simulink model "Diagramas_pruebas_modelo_definitivo"  (R2023b)
settings: Solver=VariableStepAuto  StartTime=0.0  StopTime=1.9  MaxStep=1e-5  RelTol=1e-3
values from neighbouring files (symbols this model uses):
  alpha_cu = 3.9 * 10^(-3)    (= 0.0039)    [parametros.m]
  b_eq = 2.1944e-5    (= 2.1944e-05)    [diagrama_polos_y_ceros_LTI.m]    (also in main.m = 2.19444444444e-05; parametros.m = 2.21527777778e-05)
  C_ts = 0.818    [parametros.m]
  J_eq = 1.9785e-5    (= 1.9785e-05)    [diagrama_polos_y_ceros_LTI.m]    (also in main.m = 1.97847222222e-05; parametros.m = 1.97847222222e-05)
  k_l = 0.25    [main.m]    (also in parametros.m)
  L_d = 6.6    [main.m]    (also in parametros.m = 0.0066)
  L_q = 5.8e-3    (= 0.0058)    [diagrama_polos_y_ceros_LTI.m]    (also in main.m = 5.8; parametros.m; variacion_de_parametros.m)
  P_p = 3    [Simulacion_Temporal_corrientesytensiones.m]    (also in diagrama_polos_y_ceros_LTI.m; main.m; parametros.m; variacion_de_parametros.m)
  r = 120.0    (= 120)    [diagrama_polos_y_ceros_LTI.m]    (also in main.m; parametros.m)
  R_sref = 1.02    [parametros.m]
  R_tsamb = 146.7    [parametros.m]
  T_sref = 20    [parametros.m]
libraries: SignalEditorBlockLib x2
settings Model: Creator=nicol  LastModifiedBy=Julya

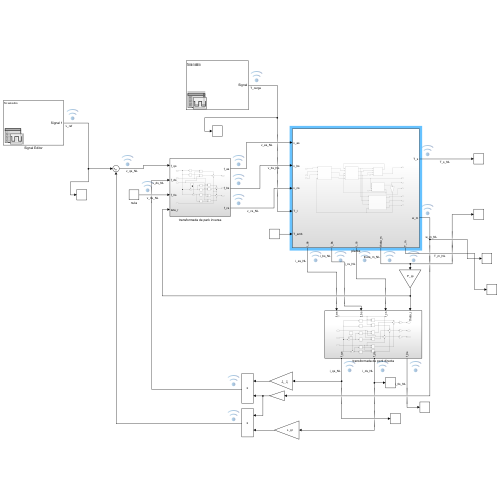
[thumbnail: Simulink's stored preview of the top-level diagram]
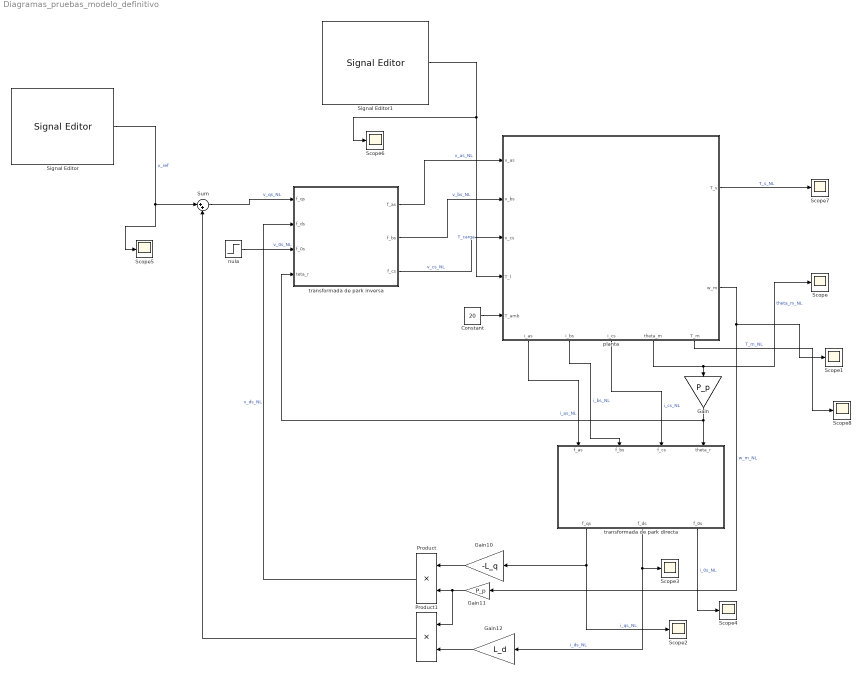
== system Diagramas_pruebas_modelo_definitivo ==
  Constant : Constant  Value=20
  Gain : Gain  Gain=P_p
  Gain10 : Gain  Gain=-L_q
  Gain11 : Gain  Gain=P_p
  Gain12 : Gain  Gain=L_d
  Product : Product
  Product1 : Product
  Scope{,1..8} (9 alike) : Scope
  Signal Editor : SignalEditorBlockLib/Signal Editor  FileName=V_qs_ref.mat  ActiveScenario=Scenario  ActiveSignal=Signal 1  IsBus=off  OutputBusObjectStr=Bus: BusObject  SampleTime=0  Interpolate=off  ZeroCross=off  OutputAfterFinalValue=Setting to zero  Unit=inherit  PreserveSignalName=on  ApplySigPropsToAllScenarios=on  ApplySigPropsToAllSignals=off
  Signal Editor1 : SignalEditorBlockLib/Signal Editor  FileName=Pulso_Torque_Carga.mat  ActiveScenario=Scenario  ActiveSignal=Signal  IsBus=off  OutputBusObjectStr=Bus: BusObject  SampleTime=0  Interpolate=off  ZeroCross=off  OutputAfterFinalValue=Setting to zero  Unit=inherit  PreserveSignalName=on  ApplySigPropsToAllScenarios=on  ApplySigPropsToAllSignals=off
  Sum : Sum  Inputs=|++
  nula : Step  Time=0  After=0  SampleTime=0
  planta : Subsystem
      settings: PortSchema="{\"entries\":[{\"content\":{\"sides\":[{\"content\":{\"connectorIds\":[\"In1\",\"In2\",\"In3\",\"In4\",\"In5\"]},\"type\":\"ConnectorPlacement.EquallySpacedRectSide\",\"uuid\":\"2cf6e661-0430-4ac8-a786-dfa08ffeeb54\"},{\"content\":{\"connectorIds\":[\"Out1\",\"Out2\"],\"side\":\"RIGHT\"},\"type\":\"ConnectorPlacement.EquallySpacedRectSide\",\"uuid\":\"d76a4f35-fdbe-4ab9-8127-b0e4effef06c\"},{\"content\":{\"side\":\"TOP\"},\"type\":\"ConnectorPlacement.EquallySpacedRectSide\",\"uuid\":\"e280a4ce-2875-4086-a9ae-a62a28e40d14\"},{\"content\":{\"connectorIds\":[\"Out3\",\"Out4\",\"Out5\",\"Out6\",\"Out7\"],\"side\":\"BOTTOM\"},\"type\":\"ConnectorPlacement.EquallySpacedRectSide\",\"uuid\":\"3ec764cb-1cf8-4a25-8759-cfccbcca4007\"}]},\"type\":\"ConnectorPlacement.EquallySpacedConnector\",\"uuid\":\"124f73b6-a202-4770-9cb1-4c0d62f02b41\"}],\"packageUris\":[\"http://schema.mathworks.com/mf0/Connector/R2020b\"],\"version\":\"1.0\"}"
  transformada de park directa : Subsystem
  transformada de park inversa : Subsystem
  wires:
  planta/3(i_as) -> transformada de park directa/1(f_as)  "i_as_NL"
  planta/4(i_bs) -> transformada de park directa/2(f_bs)  "i_bs_NL"
  planta/5(i_cs) -> transformada de park directa/3(f_cs)  "i_cs_NL"
  planta/6(theta_m) -> Gain/1, Scope/1  "theta_m_NL"
  Gain/1 -> transformada de park inversa/4(teta_r), transformada de park directa/4(theta_r)
  Gain12/1 -> Product1/2
  Gain11/1 -> Product1/1, Product/2
  Gain10/1 -> Product/1
  transformada de park directa/1(f_qs) -> Scope2/1, Gain10/1  "i_qs_NL"
  planta/2(w_m) -> Scope1/1, Gain11/1  "w_m_NL"
  transformada de park directa/2(f_ds) -> Scope3/1, Gain12/1  "i_ds_NL"
  Product/1 -> transformada de park inversa/2(f_ds)  "v_ds_NL"
  Product1/1 -> Sum/2
  Sum/1 -> transformada de park inversa/1(f_qs)  "v_qs_NL"
  transformada de park inversa/1(f_as) -> planta/1(v_as)  "v_as_NL"
  transformada de park inversa/2(f_bs) -> planta/2(v_bs)  "v_bs_NL"
  transformada de park inversa/3(f_cs) -> planta/3(v_cs)  "v_cs_NL"
  Signal Editor/1 -> Scope5/1, Sum/1  "v_ref"
  Signal Editor1/1 -> Scope6/1, planta/4(T_l)  "T_carga"
  transformada de park directa/3(f_0s) -> Scope4/1  "i_0s_NL"
  planta/1(T_s) -> Scope7/1  "T_s_NL"
  Constant/1 -> planta/5(T_amb)
  planta/7(T_m) -> Scope8/1  "T_m_NL"
  nula/1 -> transformada de park inversa/3(f_0s)  "v_0s_NL"

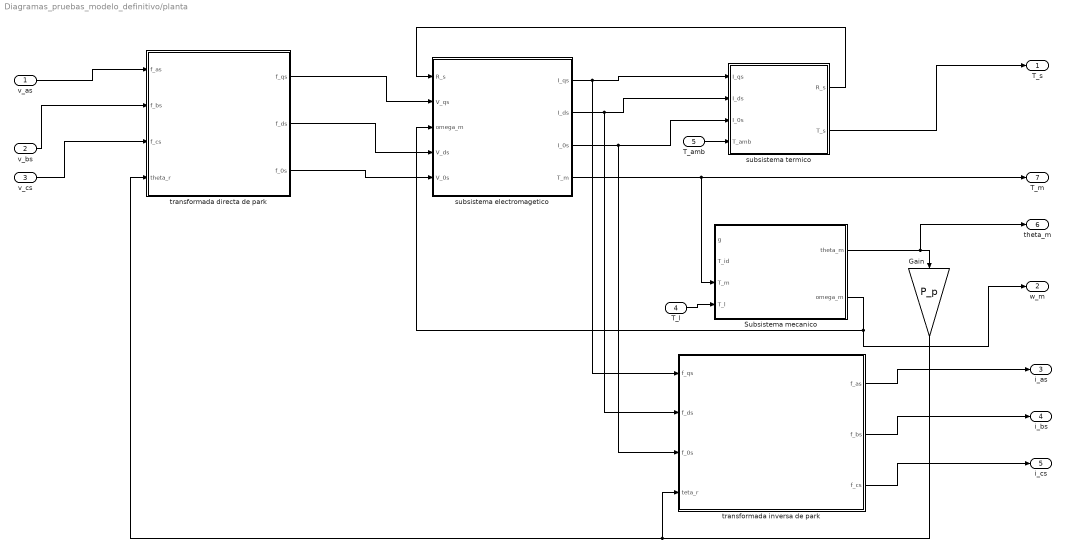
== system Diagramas_pruebas_modelo_definitivo/planta ==
  v_as : Inport
  v_bs : Inport  Port=2
  v_cs : Inport  Port=3
  T_l : Inport  Port=4
  T_amb : Inport  Port=5
  Gain : Gain  Gain=P_p
  Subsistema mecanico : Subsystem
  subsistema electromagetico : Subsystem
  subsistema termico : Subsystem
  transformada directa de park : Subsystem
  transformada inversa de park : Subsystem
  T_s : Outport
  w_m : Outport  Port=2
  i_as : Outport  Port=3
  i_bs : Outport  Port=4
  i_cs : Outport  Port=5
  theta_m : Outport  Port=6
  T_m : Outport  Port=7
  wires:
  transformada directa de park/1(f_qs) -> subsistema electromagetico/2(V_qs)
  transformada directa de park/2(f_ds) -> subsistema electromagetico/4(V_ds)
  transformada directa de park/3(f_0s) -> subsistema electromagetico/5(V_0s)
  subsistema termico/1(R_s) -> subsistema electromagetico/1(R_s)
  subsistema electromagetico/1(I_qs) -> transformada inversa de park/1(f_qs), subsistema termico/1(I_qs)
  subsistema electromagetico/2(I_ds) -> transformada inversa de park/2(f_ds), subsistema termico/2(I_ds)
  subsistema electromagetico/3(I_0s) -> transformada inversa de park/3(f_0s), subsistema termico/3(I_0s)
  subsistema electromagetico/4(T_m) -> T_m/1, Subsistema mecanico/3(T_m)
  Subsistema mecanico/2(omega_m) -> w_m/1, subsistema electromagetico/3(omega_m)
  Subsistema mecanico/1(theta_m) -> theta_m/1, Gain/1
  Gain/1 -> transformada directa de park/4(theta_r), transformada inversa de park/4(teta_r)
  v_as/1 -> transformada directa de park/1(f_as)
  v_bs/1 -> transformada directa de park/2(f_bs)
  v_cs/1 -> transformada directa de park/3(f_cs)
  subsistema termico/2(T_s) -> T_s/1
  transformada inversa de park/1(f_as) -> i_as/1
  transformada inversa de park/2(f_bs) -> i_bs/1
  transformada inversa de park/3(f_cs) -> i_cs/1
  T_l/1 -> Subsistema mecanico/4(T_l)
  T_amb/1 -> subsistema termico/4(T_amb)

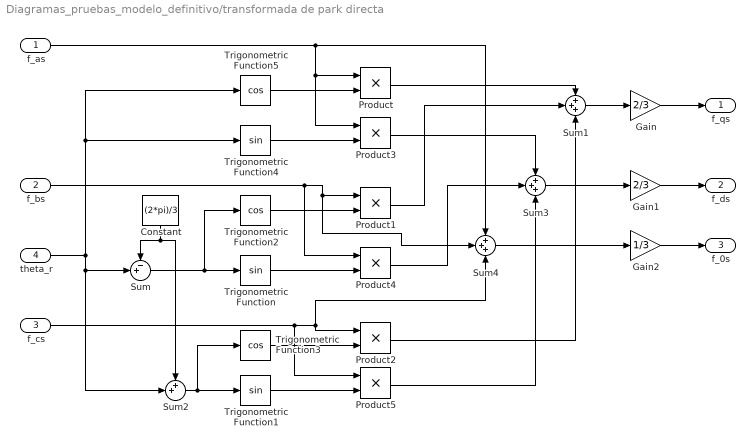
== system Diagramas_pruebas_modelo_definitivo/transformada de park directa ==
  f_as : Inport
  f_bs : Inport  Port=2
  f_cs : Inport  Port=3
  theta_r : Inport  Port=4
  Constant : Constant  Value=(2*pi)/3
  Gain : Gain  Gain=2/3
  Gain1 : Gain  Gain=2/3
  Gain2 : Gain  Gain=1/3
  Product{,1..5} (6 alike) : Product
  Sum : Sum  Inputs=-+|
  Sum1 : Sum  Inputs=+++
  Sum2 : Sum  Inputs=++|
  Sum3 : Sum  Inputs=+++
  Sum4 : Sum  Inputs=+++
  Trigonometric Function : Trigonometry
  Trigonometric Function1 : Trigonometry
  Trigonometric Function2 : Trigonometry  Operator=cos
  Trigonometric Function3 : Trigonometry  Operator=cos
  Trigonometric Function4 : Trigonometry
  Trigonometric Function5 : Trigonometry  Operator=cos
  f_qs : Outport
  f_ds : Outport  Port=2
  f_0s : Outport  Port=3
  wires:
  Sum4/1 -> Gain2/1
  Sum3/1 -> Gain1/1
  Trigonometric Function3/1 -> Product2/2
  Gain1/1 -> f_ds/1
  Gain2/1 -> f_0s/1
  f_bs/1 -> Sum4/2, Product1/1, Product4/1
  f_as/1 -> Sum4/1, Product3/1, Product/1
  Trigonometric Function2/1 -> Product1/2
  Trigonometric Function4/1 -> Product3/2
  Trigonometric Function/1 -> Product4/2
  Sum/1 -> Trigonometric Function/1, Trigonometric Function2/1
  Gain/1 -> f_qs/1
  Product5/1 -> Sum3/3
  Product3/1 -> Sum3/1
  Trigonometric Function1/1 -> Product5/2
  Product4/1 -> Sum3/2
  Product/1 -> Sum1/1
  theta_r/1 -> Sum2/2, Sum/2, Trigonometric Function5/1, Trigonometric Function4/1
  Constant/1 -> Sum/1, Sum2/1
  Sum2/1 -> Trigonometric Function3/1, Trigonometric Function1/1
  Sum1/1 -> Gain/1
  Product1/1 -> Sum1/2
  f_cs/1 -> Sum4/3, Product2/1, Product5/1
  Product2/1 -> Sum1/3
  Trigonometric Function5/1 -> Product/2

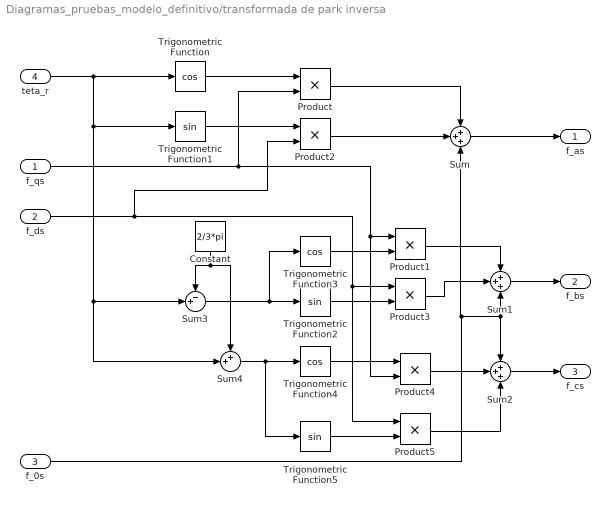
== system Diagramas_pruebas_modelo_definitivo/transformada de park inversa ==
  f_qs : Inport
  f_ds : Inport  Port=2
  f_0s : Inport  Port=3
  teta_r : Inport  Port=4
  Constant : Constant  Value=2/3*pi
  Product{,1..5} (6 alike) : Product
  Sum : Sum  Inputs=+++
  Sum1 : Sum  Inputs=+++
  Sum2 : Sum  Inputs=+++
  Sum3 : Sum  Inputs=-+|
  Sum4 : Sum  Inputs=++|
  Trigonometric Function : Trigonometry  Operator=cos
  Trigonometric Function1 : Trigonometry
  Trigonometric Function2 : Trigonometry
  Trigonometric Function3 : Trigonometry  Operator=cos
  Trigonometric Function4 : Trigonometry  Operator=cos
  Trigonometric Function5 : Trigonometry
  f_as : Outport
  f_bs : Outport  Port=2
  f_cs : Outport  Port=3
  wires:
  Product1/1 -> Sum1/1
  Sum4/1 -> Trigonometric Function5/1, Trigonometric Function4/1
  Sum2/1 -> f_cs/1
  Product2/1 -> Sum/2
  Trigonometric Function/1 -> Product/1
  Product4/1 -> Sum2/2
  Sum1/1 -> f_bs/1
  Trigonometric Function3/1 -> Product1/2
  Trigonometric Function5/1 -> Product5/2
  Product/1 -> Sum/1
  Sum3/1 -> Trigonometric Function3/1, Trigonometric Function2/1
  Trigonometric Function4/1 -> Product4/1
  f_0s/1 -> Sum/3, Sum2/1, Sum1/3
  Trigonometric Function2/1 -> Product3/2
  f_qs/1 -> Product1/1, Product4/2, Product/2
  teta_r/1 -> Sum4/2, Sum3/2, Trigonometric Function1/1, Trigonometric Function/1
  Product3/1 -> Sum1/2
  Trigonometric Function1/1 -> Product2/1
  f_ds/1 -> Product3/1, Product5/1, Product2/2
  Product5/1 -> Sum2/3
  Constant/1 -> Sum4/1, Sum3/1
  Sum/1 -> f_as/1

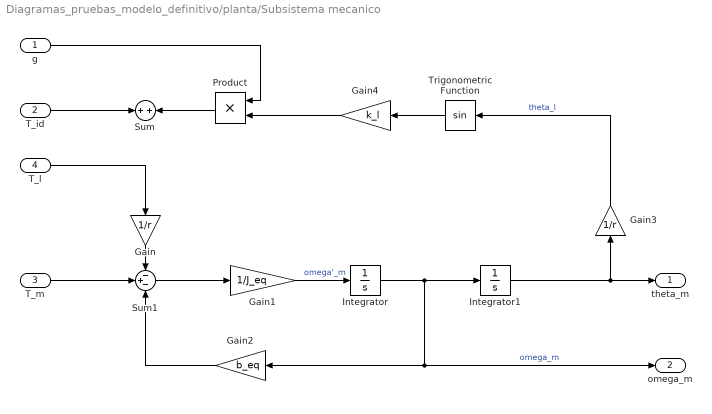
== system Diagramas_pruebas_modelo_definitivo/planta/Subsistema mecanico ==
  g : Inport
  T_id : Inport  Port=2
  T_m : Inport  Port=3
  T_l : Inport  Port=4
  Gain : Gain  Gain=1/r
  Gain1 : Gain  Gain=1/J_eq
  Gain2 : Gain  Gain=b_eq
  Gain3 : Gain  Gain=1/r
  Gain4 : Gain  Gain=k_l
  Integrator : Integrator
  Integrator1 : Integrator
  Product : Product
  Sum : Sum
  Sum1 : Sum  Inputs=-+-
  Trigonometric Function : Trigonometry
  theta_m : Outport
  omega_m : Outport  Port=2
  wires:
  Sum1/1 -> Gain1/1
  Gain1/1 -> Integrator/1  "omega'_m"
  g/1 -> Product/1
  T_m/1 -> Sum1/2
  T_id/1 -> Sum/1
  Gain2/1 -> Sum1/3
  Gain/1 -> Sum1/1
  Integrator/1 -> Integrator1/1, omega_m/1, Gain2/1  "omega_m"
  Product/1 -> Sum/2
  Gain3/1 -> Trigonometric Function/1  "theta_l"
  Trigonometric Function/1 -> Gain4/1
  Integrator1/1 -> theta_m/1, Gain3/1
  Gain4/1 -> Product/2
  T_l/1 -> Gain/1

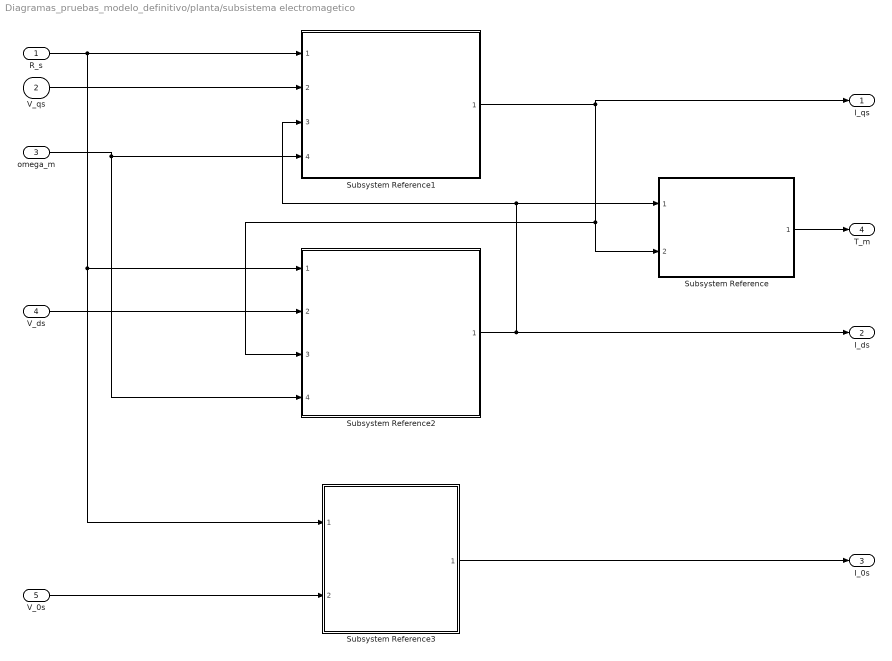
== system Diagramas_pruebas_modelo_definitivo/planta/subsistema electromagetico ==
  R_s : Inport
  V_qs : Inport  Port=2
  omega_m : Inport  Port=3
  V_ds : Inport  Port=4
  V_0s : Inport  Port=5
  Subsystem Reference : Subsystem  ReferencedSubsystem=subsistema_magnetico_estator
  Subsystem Reference1 : Subsystem  ReferencedSubsystem=subsistema_electrico_corriente_I_qs
  Subsystem Reference2 : Subsystem  ReferencedSubsystem=subsistema_electrico_corriente_I_ds
  Subsystem Reference3 : Subsystem  ReferencedSubsystem=subsistema_electrico_corriente_I_0s
  I_qs : Outport
  I_ds : Outport  Port=2
  I_0s : Outport  Port=3
  T_m : Outport  Port=4
  wires:
  Subsystem Reference/1 -> T_m/1
  V_ds/1 -> Subsystem Reference2/2
  omega_m/1 -> Subsystem Reference1/4, Subsystem Reference2/4
  V_0s/1 -> Subsystem Reference3/2
  V_qs/1 -> Subsystem Reference1/2
  Subsystem Reference1/1 -> I_qs/1, Subsystem Reference/2, Subsystem Reference2/3
  Subsystem Reference2/1 -> Subsystem Reference1/3, Subsystem Reference/1, I_ds/1
  Subsystem Reference3/1 -> I_0s/1
  R_s/1 -> Subsystem Reference1/1, Subsystem Reference2/1, Subsystem Reference3/1

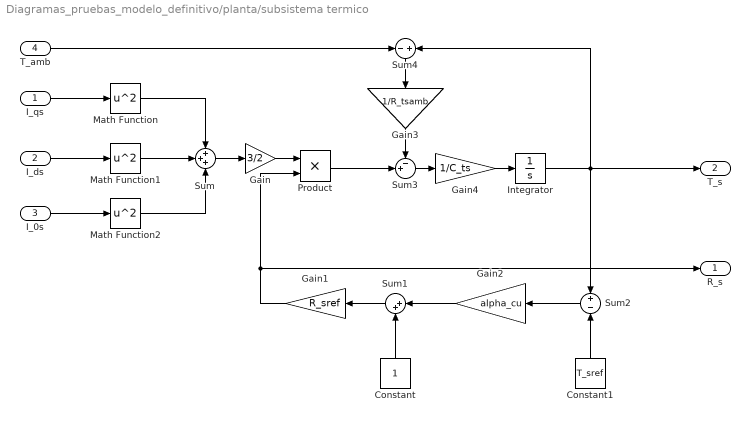
== system Diagramas_pruebas_modelo_definitivo/planta/subsistema termico ==
  I_qs : Inport
  I_ds : Inport  Port=2
  I_0s : Inport  Port=3
  T_amb : Inport  Port=4
  Constant : Constant
  Constant1 : Constant  Value=T_sref
  Gain : Gain  Gain=3/2
  Gain1 : Gain  Gain=R_sref
  Gain2 : Gain  Gain=alpha_cu
  Gain3 : Gain  Gain=1/R_tsamb
  Gain4 : Gain  Gain=1/C_ts
  Integrator : Integrator  InitialCondition=20
  Math Function : Math  Operator=square
  Math Function1 : Math  Operator=square
  Math Function2 : Math  Operator=square
  Product : Product
  Sum : Sum  Inputs=+++
  Sum1 : Sum  Inputs=|++
  Sum2 : Sum  Inputs=+|-
  Sum3 : Sum  Inputs=-+|
  Sum4 : Sum  Inputs=-|+
  R_s : Outport
  T_s : Outport  Port=2
  wires:
  Gain1/1 -> Product/2, R_s/1
  Constant1/1 -> Sum2/2
  Math Function/1 -> Sum/1
  Gain2/1 -> Sum1/1
  Integrator/1 -> Sum2/1, T_s/1, Sum4/2
  Constant/1 -> Sum1/2
  Gain3/1 -> Sum3/1
  T_amb/1 -> Sum4/1
  Product/1 -> Sum3/2
  Sum3/1 -> Gain4/1
  Gain/1 -> Product/1
  Sum2/1 -> Gain2/1
  I_0s/1 -> Math Function2/1
  Gain4/1 -> Integrator/1
  I_ds/1 -> Math Function1/1
  Sum4/1 -> Gain3/1
  Math Function1/1 -> Sum/2
  Sum/1 -> Gain/1
  I_qs/1 -> Math Function/1
  Sum1/1 -> Gain1/1
  Math Function2/1 -> Sum/3

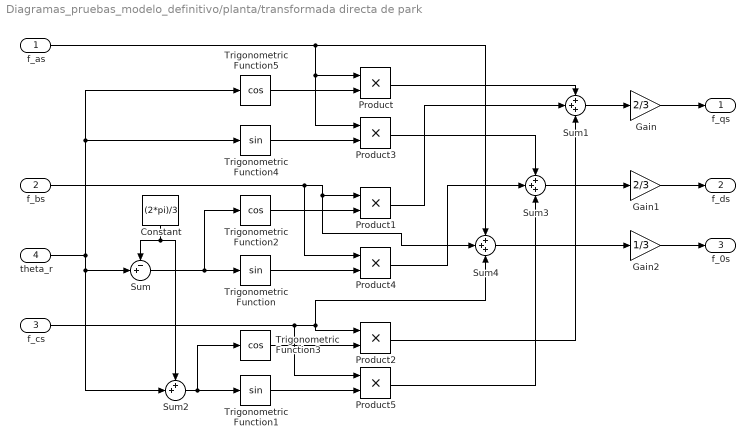
== system Diagramas_pruebas_modelo_definitivo/planta/transformada directa de park ==
  f_as : Inport
  f_bs : Inport  Port=2
  f_cs : Inport  Port=3
  theta_r : Inport  Port=4
  Constant : Constant  Value=(2*pi)/3
  Gain : Gain  Gain=2/3
  Gain1 : Gain  Gain=2/3
  Gain2 : Gain  Gain=1/3
  Product{,1..5} (6 alike) : Product
  Sum : Sum  Inputs=-+|
  Sum1 : Sum  Inputs=+++
  Sum2 : Sum  Inputs=++|
  Sum3 : Sum  Inputs=+++
  Sum4 : Sum  Inputs=+++
  Trigonometric Function : Trigonometry
  Trigonometric Function1 : Trigonometry
  Trigonometric Function2 : Trigonometry  Operator=cos
  Trigonometric Function3 : Trigonometry  Operator=cos
  Trigonometric Function4 : Trigonometry
  Trigonometric Function5 : Trigonometry  Operator=cos
  f_qs : Outport
  f_ds : Outport  Port=2
  f_0s : Outport  Port=3
  wires:
  Sum4/1 -> Gain2/1
  Sum3/1 -> Gain1/1
  Trigonometric Function3/1 -> Product2/2
  Gain1/1 -> f_ds/1
  Gain2/1 -> f_0s/1
  f_bs/1 -> Sum4/2, Product1/1, Product4/1
  f_as/1 -> Sum4/1, Product3/1, Product/1
  Trigonometric Function2/1 -> Product1/2
  Trigonometric Function4/1 -> Product3/2
  Trigonometric Function/1 -> Product4/2
  Sum/1 -> Trigonometric Function/1, Trigonometric Function2/1
  Gain/1 -> f_qs/1
  Product5/1 -> Sum3/3
  Product3/1 -> Sum3/1
  Trigonometric Function1/1 -> Product5/2
  Product4/1 -> Sum3/2
  Product/1 -> Sum1/1
  theta_r/1 -> Sum2/2, Sum/2, Trigonometric Function5/1, Trigonometric Function4/1
  Constant/1 -> Sum/1, Sum2/1
  Sum2/1 -> Trigonometric Function3/1, Trigonometric Function1/1
  Sum1/1 -> Gain/1
  Product1/1 -> Sum1/2
  f_cs/1 -> Sum4/3, Product2/1, Product5/1
  Product2/1 -> Sum1/3
  Trigonometric Function5/1 -> Product/2

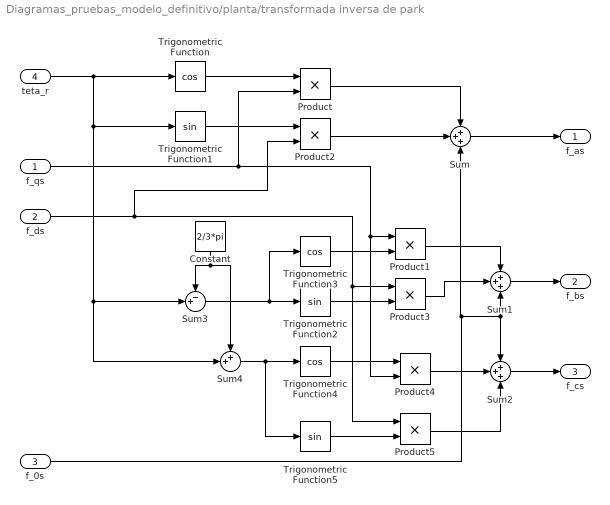
== system Diagramas_pruebas_modelo_definitivo/planta/transformada inversa de park ==
  f_qs : Inport
  f_ds : Inport  Port=2
  f_0s : Inport  Port=3
  teta_r : Inport  Port=4
  Constant : Constant  Value=2/3*pi
  Product{,1..5} (6 alike) : Product
  Sum : Sum  Inputs=+++
  Sum1 : Sum  Inputs=+++
  Sum2 : Sum  Inputs=+++
  Sum3 : Sum  Inputs=-+|
  Sum4 : Sum  Inputs=++|
  Trigonometric Function : Trigonometry  Operator=cos
  Trigonometric Function1 : Trigonometry
  Trigonometric Function2 : Trigonometry
  Trigonometric Function3 : Trigonometry  Operator=cos
  Trigonometric Function4 : Trigonometry  Operator=cos
  Trigonometric Function5 : Trigonometry
  f_as : Outport
  f_bs : Outport  Port=2
  f_cs : Outport  Port=3
  wires:
  Product1/1 -> Sum1/1
  Sum4/1 -> Trigonometric Function5/1, Trigonometric Function4/1
  Sum2/1 -> f_cs/1
  Product2/1 -> Sum/2
  Trigonometric Function/1 -> Product/1
  Product4/1 -> Sum2/2
  Sum1/1 -> f_bs/1
  Trigonometric Function3/1 -> Product1/2
  Trigonometric Function5/1 -> Product5/2
  Product/1 -> Sum/1
  Sum3/1 -> Trigonometric Function3/1, Trigonometric Function2/1
  Trigonometric Function4/1 -> Product4/1
  f_0s/1 -> Sum/3, Sum2/1, Sum1/3
  Trigonometric Function2/1 -> Product3/2
  f_qs/1 -> Product1/1, Product4/2, Product/2
  teta_r/1 -> Sum4/2, Sum3/2, Trigonometric Function1/1, Trigonometric Function/1
  Product3/1 -> Sum1/2
  Trigonometric Function1/1 -> Product2/1
  f_ds/1 -> Product3/1, Product5/1, Product2/2
  Product5/1 -> Sum2/3
  Constant/1 -> Sum4/1, Sum3/1
  Sum/1 -> f_as/1
